simulink model "quadrotor_mellinger"  (R2024a)
settings: Solver=FixedStepAuto  StartTime=0.0  StopTime=30  FixedStep=0.0041667  RelTol=1e-3
values from neighbouring files (symbols this model uses):
  air_density = 1.229    [main2.m]    (also in param_set.m)
  bias_acc = task_bias_acc(task_id)    [main2.m]    (also in param_set.m = (-1+2*rand)*20/1000)
  bias_gyro = task_bias_gyro(task_id)    [main2.m]    (also in param_set.m = (-1+2*rand)*1)
  cf_mass = ori_mass + mass_payload    (= 0.027)    [main2.m]    (also in param_set.m)
  complex_pulse = ismember(task_id, [7, 8])    [main2.m]    (also in param_set.m = 0)
  delay_coef_acc = 100    [main2.m]    (also in param_set.m)
  delay_coef_gyro = 230    [main2.m]    (also in param_set.m)
  delay_coef_motor = 50    [main2.m]    (also in param_set.m)
  g = 9.81    [main2.m]    (also in param_set.m)
  goal_pos = task_goal_pos(task_id, :)    [main2.m]    (also in param_set.m = [0, 0.01, 1])
  GRAVITY_FORCE = g * cf_mass    (= 0.26487)    [main2.m]    (also in param_set.m)
  Kd_lin = data_struct.Kd_lin    [generate_mat_files.m]    (also in main2.m = [0.3114; 0.3114; 1.1489]; param_set.m = [0.3114; 0.3114; 1.1489])
  Ki_lin = data_struct.Ki_lin    [generate_mat_files.m]    (also in main2.m = [0.0027; 0.0027; 0.2500]; param_set.m = [0.0027; 0.0027; 0.2500])
  Ki_rot = data_struct.Ki_rot    [generate_mat_files.m]    (also in main2.m = [-1.2303; -1.2303; 494.9237]; param_set.m = [-1.2303; -1.2303; 494.9237])
  Kp_lin = data_struct.Kp_lin    [generate_mat_files.m]    (also in main2.m = [0.4319; 0.4319; 2.5857]; param_set.m = [0.4319; 0.4319; 2.5857])
  Kr_rot = data_struct.Kr_rot    [generate_mat_files.m]    (also in main2.m = [70000.0; 70000.0; 60000.0]; param_set.m = [70000.0; 70000.0; 60000.0])
  Kw_rot = data_struct.Kw_rot    [generate_mat_files.m]    (also in main2.m = [20000.0; 20000.0; 12000.0]; param_set.m = [20000.0; 20000.0; 12000.0])
  MassThrust = 132000    [main2.m]    (also in param_set.m)
  Matrix_rpm_Ftau = [ ... (first row only)    [main2.m]    (also in param_set.m)
  MaxPWM = 65535    [main2.m]    (also in param_set.m)
  measure_switch = mod(task_id, 2) == 0    [main2.m]    (also in param_set.m = 0)
  MIXER_MATRIX = [ ... (first row only)    [main2.m]    (also in param_set.m = [      -0.5, -0.5, -1.0;      -0.5,  0.5,  1.0;       0.5,  )
  pressure = 101.3e3    (= 101300)    [main2.m]    (also in param_set.m)
  PWM2RPM_CONST = 4070.3    [main2.m]    (also in param_set.m)
  PWM2RPM_SCALE = 0.2685    [main2.m]    (also in param_set.m)
  Speed_Sound = 340    [main2.m]    (also in param_set.m)
  T_flip = eye(3)    [main2.m]    (also in param_set.m = [1,  0,  0;            0,  1,  0;            0,  0,  1])
  target_x_c = [1; 0; 0]    [main2.m]    (also in param_set.m)
  UINT16_MAX = 65535    [main2.m]    (also in param_set.m)
  Wind_phi = 0    [main2.m]    (also in param_set.m)
  Wind_theta = 0    [main2.m]    (also in param_set.m)
  WorkTemperature = 25    [main2.m]    (also in param_set.m)
undefined symbols (not defined in the file or in its folder): DiscIntNeverNeededParam
libraries: simulink x12, slctrl_linear x3, sharedtransform x2, matrix_library x2, dspmathops x2, shared6dof x1
settings Model: Creator=cxk  LastModifiedBy=18065
settings OptimizationCC: ReuseModelBlockBuffer=off
settings RTWCC: GPUComputeCapability=3.5

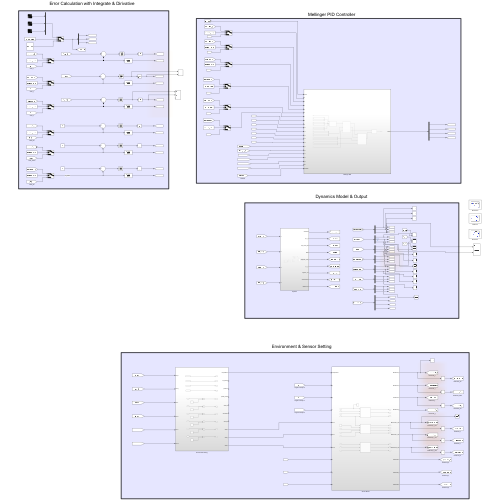
[thumbnail: Simulink's stored preview of the top-level diagram]
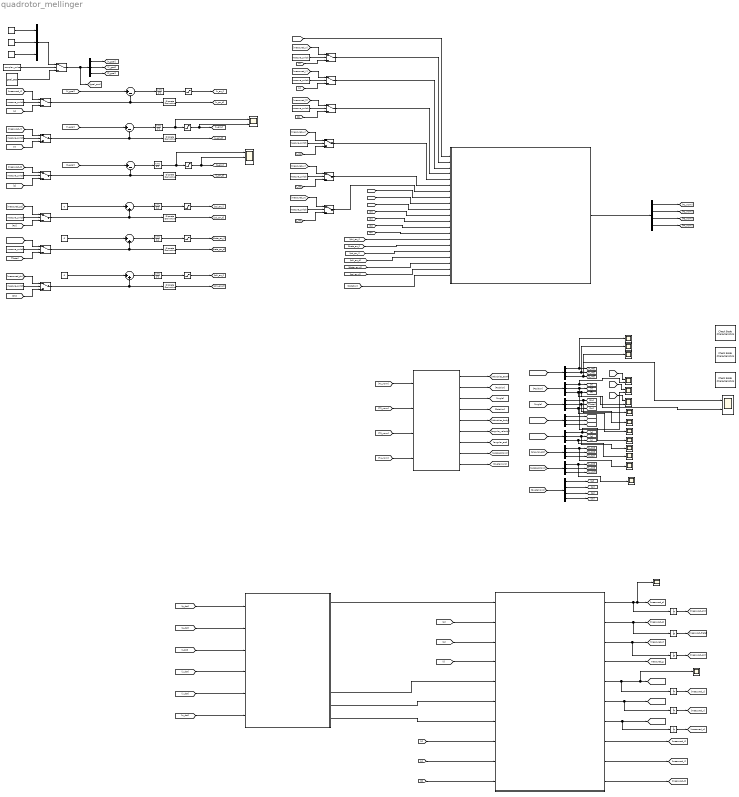
== system quadrotor_mellinger ==
  note: Mellinger PID Controller
  note: T1_norm
  note: Dynamics Model & Output
  note: Environment & Sensor Setting
  note: Error Calculation with Integrate & Dirivative
  Bode Plot : slctrl_linear/Check Bode  Characteristics  InstantiateOnLoad=on  SaveOperatingPoints=off  LinearizationIOs={'/Dynamic/From6', 1, 'outin', 'on', ''}  LinearizeAt=SnapshotTimes  SnapshotTimes=[0]  TriggerType=rising  SampleTime=auto  RateConversionMethod=zoh  PreWarpFreq=10  UseExactDelayModel=off  UseFullBlockNameLabels=off  UseBusSignalLabels=off  enabled=on  stopWhenAssertionFail=off  export=off  ViewDlgPos=[631 545 942 590]  OpenViewOnLoad=on  LaunchViewOnOpen=off  FrequencyUnits=rad/s  MagnitudeUnits=dB  PhaseUnits=deg  TimeUnits=seconds  EnableUpperBound=off  UpperBoundFrequencies=[]  UpperBoundMagnitudes=[]  EnableLowerBound=off  LowerBoundFrequencies=[]  LowerBoundMagnitudes=[]
      settings: LibrarySourceBlock=slctrlblks/Linear Analysis Plots/Bode Plot  SaveToWorkspace=off  SaveName=sys
  Bode Plot1 : slctrl_linear/Check Bode  Characteristics  InstantiateOnLoad=on  SaveOperatingPoints=off  LinearizationIOs={'/Dynamic/From6', 1, 'outin', 'on', ''}  LinearizeAt=SnapshotTimes  SnapshotTimes=[0]  TriggerType=rising  SampleTime=auto  RateConversionMethod=zoh  PreWarpFreq=10  UseExactDelayModel=off  UseFullBlockNameLabels=off  UseBusSignalLabels=off  enabled=on  stopWhenAssertionFail=off  export=off  ViewDlgPos=[1581 545.666666666667 957 589.333333333333]  OpenViewOnLoad=on  LaunchViewOnOpen=off  FrequencyUnits=rad/s  MagnitudeUnits=dB  PhaseUnits=deg  TimeUnits=seconds  EnableUpperBound=off  UpperBoundFrequencies=[]  UpperBoundMagnitudes=[]  EnableLowerBound=off  LowerBoundFrequencies=[]  LowerBoundMagnitudes=[]
      settings: LibrarySourceBlock=slctrlblks/Linear Analysis Plots/Bode Plot  SaveToWorkspace=off  SaveName=sys
  Bode Plot3 : slctrl_linear/Check Bode  Characteristics  InstantiateOnLoad=on  SaveOperatingPoints=off  LinearizationIOs={'/Dynamic/Sum', 1, 'outin', 'on', ''}  LinearizeAt=SnapshotTimes  SnapshotTimes=[0]  TriggerType=rising  SampleTime=auto  RateConversionMethod=zoh  PreWarpFreq=10  UseExactDelayModel=off  UseFullBlockNameLabels=off  UseBusSignalLabels=off  enabled=on  stopWhenAssertionFail=off  export=off  ViewDlgPos=[687.666666666667 401 778.666666666667 390]  OpenViewOnLoad=on  LaunchViewOnOpen=off  FrequencyUnits=rad/s  MagnitudeUnits=dB  PhaseUnits=deg  TimeUnits=seconds  EnableUpperBound=off  UpperBoundFrequencies=[]  UpperBoundMagnitudes=[]  EnableLowerBound=off  LowerBoundFrequencies=[]  LowerBoundMagnitudes=[]
      settings: LibrarySourceBlock=slctrlblks/Linear Analysis Plots/Bode Plot  SaveToWorkspace=off  SaveName=sys
  Constant : Constant  Value=goal_pos
  Constant1 : Constant  Value=0
  Constant{4..15} (12 alike) : Constant  Value=measure_switch
  Constant16 : Constant  Value=complex_pulse
  Constant2 : Constant  Value=0
  Constant3 : Constant  Value=0
  Demux{,1..4,6..7,9} (8 alike) : Demux  Outputs=3
  Demux10 : Demux
  Demux8 : Demux
  Discrete Derivative{,1..5} (6 alike) : simulink/Discrete/Discrete Derivative  gainval=1.0  ICPrevScaledInput=0.0  OutMin=[]  OutMax=[]  OutDataType=fixdt(1, 16)  OutScaling=2^-10  DoSatur=off
  Discrete-Time Integrator{,1..5} (6 alike) : DiscreteIntegrator  SampleTime=-1  ICPrevOutput=DiscIntNeverNeededParam  ICPrevScaledInput=DiscIntNeverNeededParam
  Dynamic : Subsystem
  Environment Setting : Subsystem
  Integrator{,1..5} (6 alike) : Integrator
  Mellinger PID : Subsystem
  Mux9 : Mux  Inputs=3
  Repeating Sequence1 : simulink/Sources/Repeating Sequence  rep_seq_t="[0 5 10  15 20 25 29]"  rep_seq_y=[0.05 0.05 2 2 -2 -2 0.05 ]
  Repeating Sequence2 : simulink/Sources/Repeating Sequence  rep_seq_t="[0 5 7  13 16 20 25 29]"  rep_seq_y=[0.05 0.05 1.68 1.68 -0.68 -0.68 0.05 0.05 ]
  Repeating Sequence3 : simulink/Sources/Repeating Sequence  rep_seq_t="[0 5 10  15 20 25 29]"  rep_seq_y=[0.05 0.05 2 2 -2 -2 0.05 ]
  Saturation : Saturate  UpperLimit=2  LowerLimit=-2
  Saturation1 : Saturate  UpperLimit=2  LowerLimit=-2
  Saturation2 : Saturate  UpperLimit=0.15  LowerLimit=-0.15
  Saturation3 : Saturate  UpperLimit=1  LowerLimit=-1
  Saturation4 : Saturate  UpperLimit=1  LowerLimit=-1
  Saturation5 : Saturate  UpperLimit=1  LowerLimit=-1
  Scope{,1..2,18,20} (5 alike) : Scope  NumInputPorts=2
  Scope{4..12,14,16..17,19} (13 alike) : Scope
  Scope15 : Scope  NumInputPorts=3
  Sensor Model : Subsystem
  Sum : Sum  Inputs=|+-
  Sum1 : Sum  Inputs=|+-
  Sum2 : Sum  Inputs=|+-
  Sum3 : Sum  Inputs=|++
  Sum4 : Sum  Inputs=|++
  Sum5 : Sum  Inputs=|++
  Switch{,1..11} (12 alike) : Switch  Criteria=u2 ~= 0  SaturateOnIntegerOverflow=off  InputSameDT=off
  Switch12 : Switch  Criteria=u2 > Threshold  SaturateOnIntegerOverflow=off  InputSameDT=off
  tag scope: measured_g=global
  wires:
  [T1_norm] -> Dynamic/1(In1)
  [T2_norm] -> Dynamic/2(In2)
  [T3_norm] -> Dynamic/3(In3)
  [T4_norm] -> Dynamic/4(In4)
  Dynamic/1(Velocities) -> [Velocities_earth]
  Dynamic/2(X_Y_Z) -> [Position]
  Dynamic/3(Phi_Theta_Psi) -> [Angle]
  Dynamic/4(DCM) -> [Rotation]
  Dynamic/5(Velocities_body) -> [Velocities_body]
  Dynamic/6(p_q_r) -> [angular_velocity]
  Dynamic/7(angular_acc) -> [angular_acc]
  Dynamic/8(Accelerations) -> [Accelerations]
  [Velocities_earth] -> Demux/1
  [Position] -> Demux1/1
  [Angle] -> Demux2/1
  [Accelerations] -> Demux7/1
  [angular_acc] -> Demux6/1
  [angular_velocity] -> Demux4/1
  [Velocities_body] -> Demux3/1
  Demux1/1 -> Scope/2, [X]
  Demux3/1 -> [Vx_Body]
  Demux3/2 -> [Vy_Body]
  Demux3/3 -> [Vz_Body]
  Demux6/1 -> Scope16/1, [p_dot]
  Demux6/2 -> [q_dot]
  Demux6/3 -> [r_dot]
  Demux7/1 -> Scope19/1, [u_dot]
  Demux7/2 -> [v_dot]
  Demux7/3 -> [w_dot]
  Dynamic/9(Quatenions) -> [Quatenions]
  [Quatenions] -> Demux8/1
  Demux8/1 -> [qr]
  Demux8/2 -> [qi]
  Demux9/1 -> [X_goal]
  Demux9/2 -> [Y_goal]
  Demux9/3 -> [Z_goal]
  [X_goal] -> Sum/1
  Switch1/1 -> Sum/2, Discrete Derivative2/1
  Saturation/1 -> [x_err_i]
  Discrete Derivative2/1 -> [x_err_d]
  [Y_goal] -> Sum1/1
  Switch/1 -> Sum1/2, Discrete Derivative1/1
  Discrete Derivative1/1 -> [y_err_d]
  Saturation1/1 -> Scope18/2, [y_err_i]
  [Z_goal] -> Sum2/1
  Switch2/1 -> Sum2/2, Discrete Derivative/1
  Sum2/1 -> Discrete-Time Integrator/1
  Saturation2/1 -> Scope15/2, [z_err_i]
  Saturation4/1 -> [theta_err_i]
  Constant3/1 -> Sum3/1
  Discrete Derivative4/1 -> [phi_err_d]
  Switch5/1 -> Sum3/2, Discrete Derivative4/1
  Constant2/1 -> Sum4/1
  Switch4/1 -> Sum4/2, Discrete Derivative5/1
  Discrete Derivative3/1 -> [psi_err_d]
  Saturation5/1 -> [psi_err_i]
  Switch3/1 -> Sum5/2, Discrete Derivative3/1
  Constant1/1 -> Sum5/1
  Saturation3/1 -> [phi_err_i]
  Demux10/2 -> [T2_norm]
  Demux10/4 -> [T4_norm]
  Demux10/3 -> [T3_norm]
  Switch9/1 -> Mellinger PID/2(In1)
  Switch10/1 -> Mellinger PID/3(In2)
  Switch11/1 -> Mellinger PID/4(In3)
  Switch6/1 -> Mellinger PID/5(In4)
  Switch8/1 -> Mellinger PID/6(In5)
  Switch7/1 -> Mellinger PID/7(In6)
  [x_err_i] -> Mellinger PID/8(In7)
  [y_err_i] -> Mellinger PID/9(In8)
  [z_err_i] -> Mellinger PID/10(In9)
  [qr] -> Mellinger PID/11(In10)
  [qi] -> Mellinger PID/12(In11)
  [qj] -> Mellinger PID/13(In12)
  [qk] -> Mellinger PID/14(In13)
  [phi_err_i] -> Mellinger PID/15(In14)
  [theta_err_i] -> Mellinger PID/16(In15)
  [psi_err_i] -> Mellinger PID/17(In16)
  [phi_err_d] -> Mellinger PID/18(In17)
  [theta_err_d] -> Mellinger PID/19(In18)
  [psi_err_d] -> Mellinger PID/20(In19)
  Mellinger PID/1(PWM) -> Demux10/1
  Demux10/1 -> [T1_norm]
  Demux8/3 -> [qj]
  Demux1/2 -> Scope1/2, [Y]
  Demux1/3 -> Scope2/2, Scope20/2, [Z]
  Demux2/2 -> Scope8/1, [Theta]
  Demux2/3 -> Scope9/1, [Psi]
  Demux4/3 -> Scope12/1, [r]
  Demux8/4 -> [qk]
  Demux2/1 -> [Phi], Scope4/1
  Demux4/1 -> Scope10/1, [p]
  Discrete Derivative/1 -> [z_err_d]
  Discrete-Time Integrator/1 -> Scope15/1, Saturation2/1
  Sum1/1 -> Discrete-Time Integrator1/1
  Discrete-Time Integrator1/1 -> Scope18/1, Saturation1/1
  Sum/1 -> Discrete-Time Integrator2/1
  Discrete-Time Integrator2/1 -> Saturation/1
  Sum5/1 -> Discrete-Time Integrator3/1
  Discrete-Time Integrator3/1 -> Saturation5/1
  Sum4/1 -> Discrete-Time Integrator4/1
  Discrete-Time Integrator4/1 -> Saturation4/1
  Sum3/1 -> Discrete-Time Integrator5/1
  Discrete-Time Integrator5/1 -> Saturation3/1
  Discrete Derivative5/1 -> [theta_err_d]
  Demux4/2 -> Scope11/1, [q]
  [Rotation] -> Mellinger PID/21(Rotation)
  Environment Setting/1(temperature) -> Sensor Model/1(Temperature)
  Environment Setting/8(wind x) -> Sensor Model/5(dot u)
  Environment Setting/9(wind y) -> Sensor Model/6(dot v)
  Environment Setting/10(wind z) -> Sensor Model/7(dot w)
  [p_dot] -> Environment Setting/1(dot p)
  [q_dot] -> Environment Setting/2("dot q ")
  [r_dot] -> Environment Setting/3(dot r)
  [u_dot] -> Environment Setting/4(dot u)
  [v_dot] -> Environment Setting/5(dot v)
  [w_dot] -> Environment Setting/6(dot w)
  Sensor Model/4(Measured g) -> [measured_g]
  Sensor Model/5(Measured u_dot) -> Scope17/1, [measured_u_dot], Integrator/1
  Sensor Model/6(Measured v_dot) -> Integrator1/1, [measured_v_dot]
  Sensor Model/7(Measured w_dot) -> Integrator2/1, [measured_w_dot]
  Constant4/1 -> Switch/2
  Constant5/1 -> Switch1/2
  Constant6/1 -> Switch2/2
  Constant7/1 -> Switch3/2
  Constant8/1 -> Switch4/2
  Constant9/1 -> Switch5/2
  [X] -> Switch1/3
  [Y] -> Switch/3
  [Z] -> Switch2/3
  [Psi] -> Switch3/3
  [Theta] -> Switch4/3
  [Phi] -> Switch5/3
  Constant10/1 -> Switch6/2
  [X_Vel] -> Switch6/3
  Constant11/1 -> Switch7/2
  Constant12/1 -> Switch8/2
  [Y_Vel] -> Switch8/3
  [Z_Vel] -> Switch7/3
  [measured_u] -> Switch6/1
  [measured_v] -> Switch8/1
  [measured_w] -> Switch7/1
  Sensor Model/1(Measured p) -> Integrator3/1, Scope14/1, [measured_p]
  Sensor Model/2(Measured q) -> Integrator4/1, [measured_q]
  Sensor Model/3(Measured r) -> Integrator5/1, [measured_r]
  [measured_psi] -> Switch3/1
  [measured_theta] -> Switch4/1
  [measured_phi] -> Switch5/1
  Constant13/1 -> Switch9/2
  Constant14/1 -> Switch10/2
  Constant15/1 -> Switch11/2
  [X] -> Switch9/3
  [Y] -> Switch10/3
  [Z] -> Switch11/3
  [X] -> Sensor Model/8(x)
  [Y] -> Sensor Model/9(y)
  [Z] -> Sensor Model/10(z)
  Sensor Model/8(Measured x) -> [measured_X]
  Sensor Model/9(Measured y) -> [measured_Y]
  Sensor Model/10(Measured z) -> [measured_Z]
  [measured_X] -> Switch1/1
  [measured_Y] -> Switch/1
  [measured_Z] -> Switch2/1
  [measured_X] -> Switch9/1
  [measured_Y] -> Switch10/1
  [measured_Z] -> Switch11/1
  [p] -> Sensor Model/2(p)
  [q] -> Sensor Model/3(q)
  [r] -> Sensor Model/4(r)
  Demux/1 -> Scope5/1, [X_Vel]
  Demux/2 -> Scope6/1, [Y_Vel]
  Demux/3 -> Scope20/1, [Z_Vel], Scope7/1
  Integrator3/1 -> [measured_phi]
  Integrator4/1 -> [measured_theta]
  Integrator5/1 -> [measured_psi]
  Integrator/1 -> [measured_u]
  Integrator1/1 -> [measured_v]
  Integrator2/1 -> [measured_w]
  Repeating Sequence2/1 -> Mux9/3
  [goal_pos] -> Mellinger PID/1(Goal)
  Switch12/1 -> [goal_pos], Demux9/1
  Repeating Sequence3/1 -> Mux9/1
  Repeating Sequence1/1 -> Mux9/2
  [Z_goal] -> Scope2/1
  [Y_goal] -> Scope1/1
  [X_goal] -> Scope/1
  Mux9/1 -> Switch12/1
  Constant/1 -> Switch12/3
  Constant16/1 -> Switch12/2

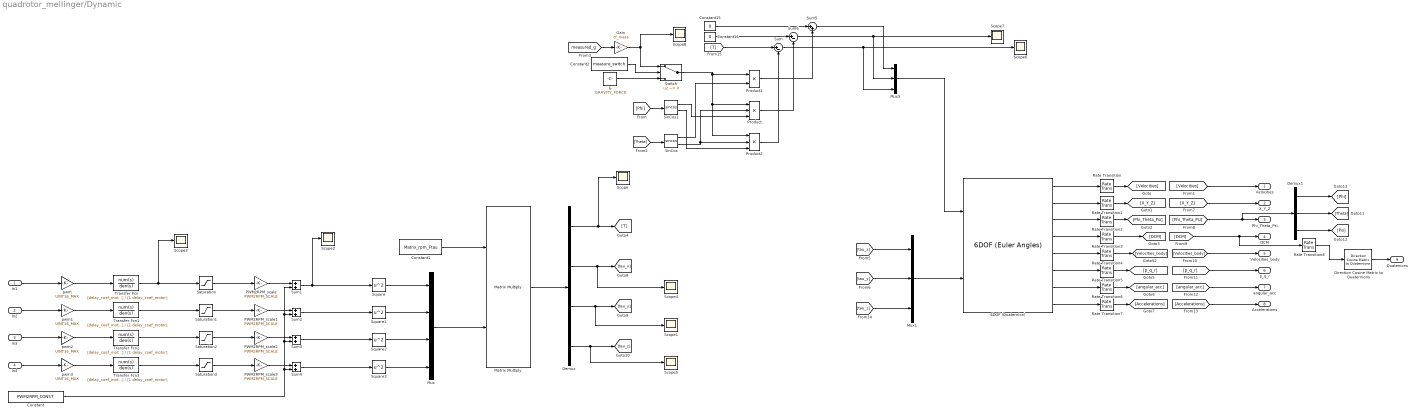
== system quadrotor_mellinger/Dynamic ==
  In1 : Inport
  In2 : Inport  Port=2
  In3 : Inport  Port=3
  In4 : Inport  Port=4
  6DOF (Quaternion) : shared6dof/6DOF (Euler Angles)  units=Metric (MKS)  mtype=Fixed  rep=Quaternion  xme_0=init_pos  Vm_0=init_vel  eul_0=init_ang  pm_0=[0 0 0]  mass_0=cf_mass  mass_e=0.5  mass_f=2.0  inertia=inertia  inertia_e=eye(3)  inertia_f=2*eye(3)  k_quat=1.0  vre_flag=on  abi_flag=off  aMode=0  xme_statename=''  Vm_statename=''  eul_statename=''  quat_statename=''  pm_statename=''  mass_statename=''
      settings: LibrarySourceBlock=aerolib6dof2/6DOF (Quaternion)
  Constant : Constant  Value=PWM2RPM_CONST
  Constant1 : Constant  Value=Matrix_rpm_Ftau
  Constant15 : Constant  Value=0
  Constant16 : Constant  Value=0
  Constant2 : Constant  Value=measure_switch
  Demux : Demux
  Demux1 : Demux  Outputs=3
  Direction Cosine Matrix to Quaternions : sharedtransform/Direction Cosine Matrix  to Quaternions  aMode=0  action=None  tolerance=eps(2)
      settings: LibrarySourceBlock=|
      | aerolibtransform2/Direction Cosine Matrix
      | to Quaternions
  G : Constant  Value=GRAVITY_FORCE
  Gain : Gain  Gain=cf_mass
  Matrix Multiply : Product  Multiplication=Matrix(*)
  Mux : Mux
  Mux1 : Mux  Inputs=3
  Mux5 : Mux  Inputs=3
  PWM2RPM_scale{,1..3} (4 alike) : Gain  Gain=PWM2RPM_SCALE
  Product : Product  Inputs=3
  Product1 : Product
  Product2 : Product  Inputs=3
  Rate Transition{,1..8} (9 alike) : RateTransition  OutPortSampleTimeOpt=Inherit  OutPortSampleTime=Ts
  Saturation{,1..3} (4 alike) : Saturate  UpperLimit=MaxPWM  LowerLimit=0
  Scope{,1..8} (9 alike) : Scope
  SinCos : Trigonometry  Operator=sincos
  SinCos1 : Trigonometry  Operator=sincos
  Square{,1..3} (4 alike) : Math  Operator=square
  Sum : Sum  Inputs=|+-
  Sum{1..4} (4 alike) : Sum
  Sum5 : Sum  Inputs=|++
  Sum6 : Sum  Inputs=|+-
  Switch : Switch  Criteria=u2 ~= 0  SaturateOnIntegerOverflow=off  InputSameDT=off
  Transfer Fcn{,1..3} (4 alike) : TransferFcn  Numerator=[delay_coef_motor]  Denominator=[1 delay_coef_motor]
  pwm{,1..3} (4 alike) : Gain  Gain=UINT16_MAX
  Velocities : Outport
  X_Y_Z : Outport  Port=2
  Phi_Theta_Psi : Outport  Port=3
  DCM : Outport  Port=4
  Velocities_body : Outport  Port=5
  p_q_r : Outport  Port=6
  angular_acc : Outport  Port=7
  Accelerations : Outport  Port=8
  Quatenions : Outport  Port=9
  wires:
  Rate Transition3/1 -> [DCM]
  Matrix Multiply/1 -> Demux/1
  Rate Transition6/1 -> [angular_acc]
  Rate Transition/1 -> [Velocities]
  [p_q_r] -> p_q_r/1
  [Velocities_body] -> Velocities_body/1
  [Phi_Theta_Psi] -> Demux1/1, Phi_Theta_Psi/1
  [tau_x] -> Mux1/1
  6DOF (Quaternion)/4 -> Rate Transition3/1
  Constant1/1 -> Matrix Multiply/1
  Demux/2 -> Scope4/1, [tau_x]
  Rate Transition5/1 -> [p_q_r]
  Rate Transition7/1 -> [Accelerations]
  Rate Transition1/1 -> [X_Y_Z]
  Rate Transition2/1 -> [Phi_Theta_Psi]
  Square1/1 -> Mux/2
  Demux/1 -> Scope/1, [T]
  Square3/1 -> Mux/4
  Mux/1 -> Matrix Multiply/2
  [Velocities] -> Velocities/1
  Rate Transition4/1 -> [Velocities_body]
  Square/1 -> Mux/1
  [DCM] -> Rate Transition8/1, DCM/1
  [X_Y_Z] -> X_Y_Z/1
  [Accelerations] -> Accelerations/1
  Demux/4 -> Scope5/1, [tau_z]
  [angular_acc] -> angular_acc/1
  Square2/1 -> Mux/3
  Demux/3 -> Scope1/1, [tau_y]
  Rate Transition8/1 -> Direction Cosine Matrix to Quaternions/1
  Direction Cosine Matrix to Quaternions/1 -> Quatenions/1
  Sum/1 -> Mux5/3, Scope6/1
  PWM2RPM_scale/1 -> Sum1/1
  Constant/1 -> Sum4/2, Sum3/2, Sum2/2, Sum1/2
  PWM2RPM_scale1/1 -> Sum2/1
  PWM2RPM_scale2/1 -> Sum3/1
  PWM2RPM_scale3/1 -> Sum4/1
  Sum2/1 -> Square1/1
  Sum1/1 -> Scope2/1, Square/1
  Sum3/1 -> Square2/1
  Sum4/1 -> Square3/1
  Saturation/1 -> PWM2RPM_scale/1
  Saturation1/1 -> PWM2RPM_scale1/1
  Saturation2/1 -> PWM2RPM_scale2/1
  Saturation3/1 -> PWM2RPM_scale3/1
  In4/1 -> pwm3/1
  pwm3/1 -> Transfer Fcn3/1
  In3/1 -> pwm2/1
  pwm2/1 -> Transfer Fcn2/1
  In2/1 -> pwm1/1
  pwm1/1 -> Transfer Fcn1/1
  In1/1 -> pwm/1
  pwm/1 -> Transfer Fcn/1
  Transfer Fcn/1 -> Scope3/1, Saturation/1
  Transfer Fcn1/1 -> Saturation1/1
  Transfer Fcn2/1 -> Saturation2/1
  Transfer Fcn3/1 -> Saturation3/1
  Demux1/2 -> [Theta]
  Demux1/3 -> [Psi]
  Demux1/1 -> [Phi]
  [Theta] -> SinCos/1
  [Phi] -> SinCos1/1
  Sum6/1 -> Mux5/2, Scope7/1
  Sum5/1 -> Mux5/1
  SinCos/1 -> Product1/2
  Product1/1 -> Sum5/2
  SinCos/2 -> Product2/2, Product/2
  SinCos1/2 -> Product2/3
  SinCos1/1 -> Product/3
  Product2/1 -> Sum/2
  Product/1 -> Sum6/2
  Constant16/1 -> Sum6/1
  Constant15/1 -> Sum5/1
  Mux1/1 -> 6DOF (Quaternion)/2
  Mux5/1 -> 6DOF (Quaternion)/1
  6DOF (Quaternion)/2 -> Rate Transition1/1
  6DOF (Quaternion)/1 -> Rate Transition/1
  6DOF (Quaternion)/3 -> Rate Transition2/1
  6DOF (Quaternion)/5 -> Rate Transition4/1
  6DOF (Quaternion)/7 -> Rate Transition6/1
  6DOF (Quaternion)/8 -> Rate Transition7/1
  [tau_y] -> Mux1/2
  [tau_z] -> Mux1/3
  G/1 -> Switch/3
  [measured_g] -> Gain/1
  Constant2/1 -> Switch/2
  [T] -> Sum/1
  Switch/1 -> Product1/1, Product2/1, Product/1
  Gain/1 -> Switch/1, Scope8/1
  6DOF (Quaternion)/6 -> Rate Transition5/1

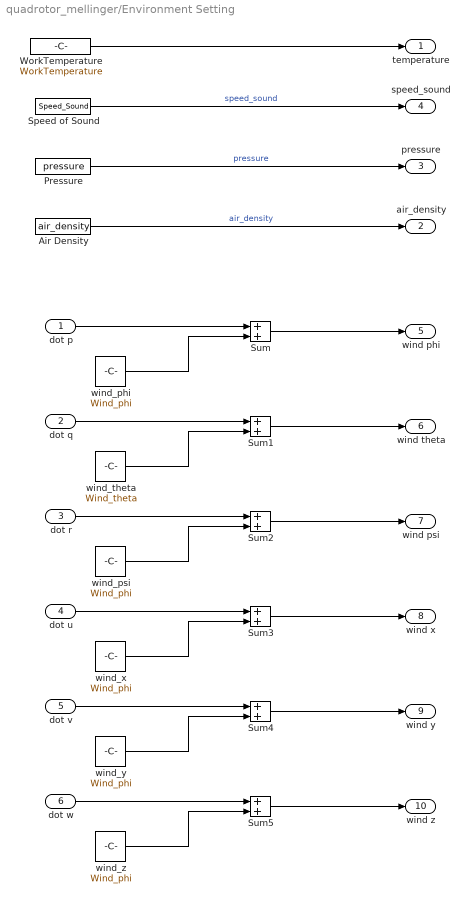
== system quadrotor_mellinger/Environment Setting ==
  dot p : Inport
  "dot q " : Inport  Port=2
  dot r : Inport  Port=3
  dot u : Inport  Port=4
  dot v : Inport  Port=5
  dot w : Inport  Port=6
  Air Density : Constant  Value=air_density
  Pressure : Constant  Value=pressure
  Speed of Sound : Constant  Value=Speed_Sound
  Sum{,1..5} (6 alike) : Sum
  WorkTemperature : Constant  Value=WorkTemperature
  wind_phi : Constant  Value=Wind_phi
  wind_psi : Constant  Value=Wind_phi
  wind_theta : Constant  Value=Wind_theta
  wind_x : Constant  Value=Wind_phi
  wind_y : Constant  Value=Wind_phi
  wind_z : Constant  Value=Wind_phi
  temperature : Outport
  air_density : Outport  Port=2
  pressure : Outport  Port=3
  speed_sound : Outport  Port=4
  wind phi : Outport  Port=5
  wind theta : Outport  Port=6
  wind psi : Outport  Port=7
  wind x : Outport  Port=8
  wind y : Outport  Port=9
  wind z : Outport  Port=10
  wires:
  Air Density/1 -> air_density/1  "air_density"
  Speed of Sound/1 -> speed_sound/1  "speed_sound"
  WorkTemperature/1 -> temperature/1
  Pressure/1 -> pressure/1  "pressure"
  dot p/1 -> Sum/1
  Sum/1 -> wind phi/1
  wind_theta/1 -> Sum1/2
  Sum1/1 -> wind theta/1
  "dot q "/1 -> Sum1/1
  wind_psi/1 -> Sum2/2
  Sum2/1 -> wind psi/1
  dot r/1 -> Sum2/1
  wind_x/1 -> Sum3/2
  Sum3/1 -> wind x/1
  dot u/1 -> Sum3/1
  wind_y/1 -> Sum4/2
  Sum4/1 -> wind y/1
  dot v/1 -> Sum4/1
  Sum5/1 -> wind z/1
  dot w/1 -> Sum5/1
  wind_phi/1 -> Sum/2
  wind_z/1 -> Sum5/2

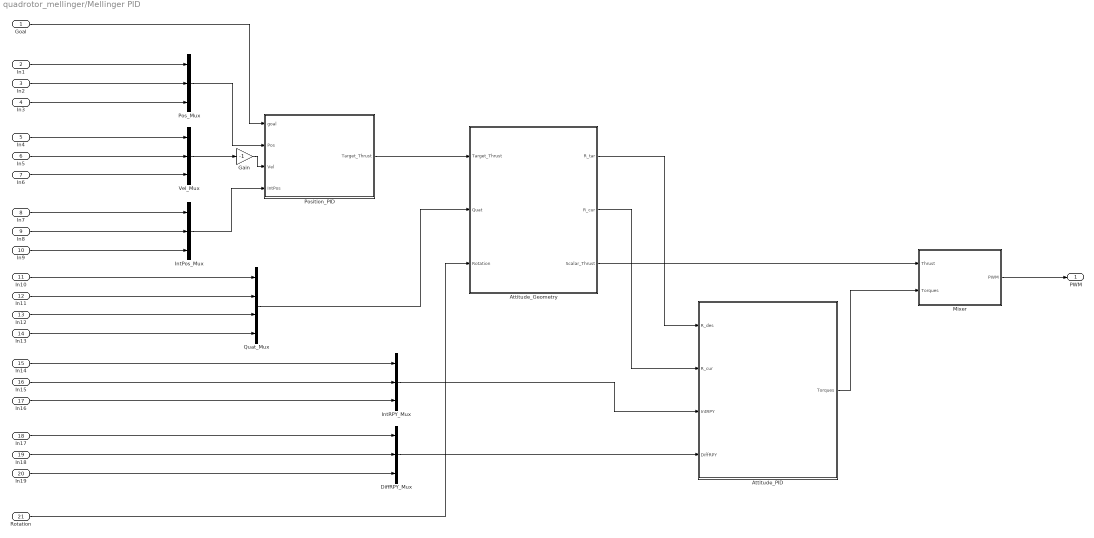
== system quadrotor_mellinger/Mellinger PID ==
  Goal : Inport
  In1 : Inport  Port=2
  In2 : Inport  Port=3
  In3 : Inport  Port=4
  In4 : Inport  Port=5
  In5 : Inport  Port=6
  In6 : Inport  Port=7
  In7 : Inport  Port=8
  In8 : Inport  Port=9
  In9 : Inport  Port=10
  In10 : Inport  Port=11
  In11 : Inport  Port=12
  In12 : Inport  Port=13
  In13 : Inport  Port=14
  In14 : Inport  Port=15
  In15 : Inport  Port=16
  In16 : Inport  Port=17
  In17 : Inport  Port=18
  In18 : Inport  Port=19
  In19 : Inport  Port=20
  Rotation : Inport  Port=21
  Attitude_Geometry : Subsystem
  Attitude_PID : Subsystem
  DiffRPY_Mux : Mux  Inputs=3
  Gain : Gain  Gain=-1
  IntPos_Mux : Mux  Inputs=3
  IntRPY_Mux : Mux  Inputs=3
  Mixer : Subsystem
  Pos_Mux : Mux  Inputs=3
  Position_PID : Subsystem
  Quat_Mux : Mux
  Vel_Mux : Mux  Inputs=3
  PWM : Outport
  wires:
  Attitude_Geometry/2(R_cur) -> Attitude_PID/2(R_cur)
  DiffRPY_Mux/1 -> Attitude_PID/4(DiffRPY)
  In17/1 -> DiffRPY_Mux/1
  In10/1 -> Quat_Mux/1
  Vel_Mux/1 -> Gain/1
  In3/1 -> Pos_Mux/3
  In9/1 -> IntPos_Mux/3
  Attitude_Geometry/3(Scalar_Thrust) -> Mixer/1(Thrust)
  In19/1 -> DiffRPY_Mux/3
  IntPos_Mux/1 -> Position_PID/4(IntPos)
  In15/1 -> IntRPY_Mux/2
  In7/1 -> IntPos_Mux/1
  In8/1 -> IntPos_Mux/2
  Quat_Mux/1 -> Attitude_Geometry/2(Quat)
  IntRPY_Mux/1 -> Attitude_PID/3(IntRPY)
  Pos_Mux/1 -> Position_PID/2(Pos)
  Attitude_PID/1(Torques) -> Mixer/2(Torques)
  Attitude_Geometry/1(R_tar) -> Attitude_PID/1(R_des)
  In11/1 -> Quat_Mux/2
  Position_PID/1(Target_Thrust) -> Attitude_Geometry/1(Target_Thrust)
  In18/1 -> DiffRPY_Mux/2
  In13/1 -> Quat_Mux/4
  In12/1 -> Quat_Mux/3
  In2/1 -> Pos_Mux/2
  In1/1 -> Pos_Mux/1
  In14/1 -> IntRPY_Mux/1
  In16/1 -> IntRPY_Mux/3
  In4/1 -> Vel_Mux/1
  In6/1 -> Vel_Mux/3
  In5/1 -> Vel_Mux/2
  Mixer/1(PWM) -> PWM/1
  Gain/1 -> Position_PID/3(Vel)
  Rotation/1 -> Attitude_Geometry/3(Rotation)
  Goal/1 -> Position_PID/1(goal)

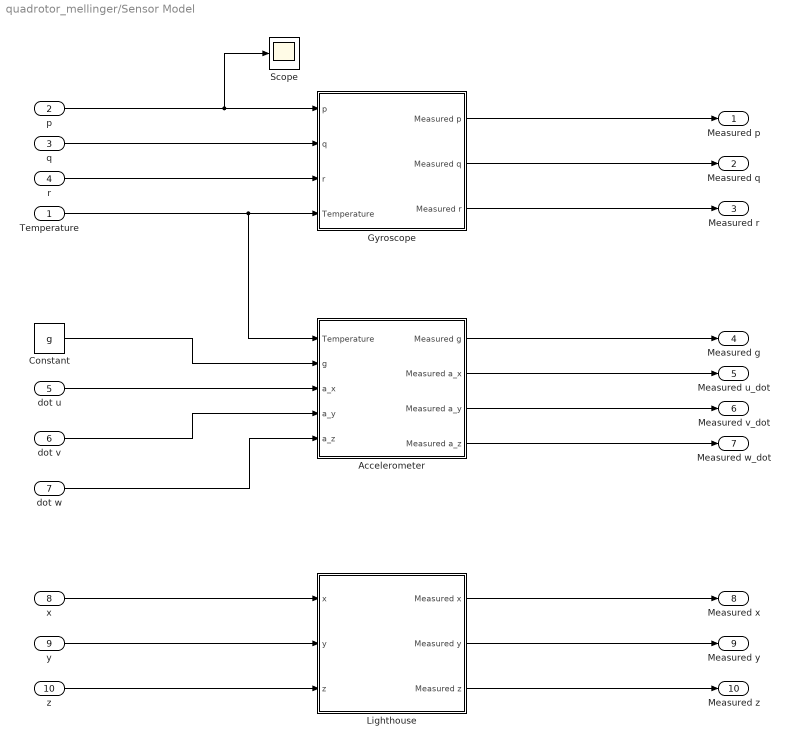
== system quadrotor_mellinger/Sensor Model ==
  Temperature : Inport
  p : Inport  Port=2
  q : Inport  Port=3
  r : Inport  Port=4
  dot u : Inport  Port=5
  dot v : Inport  Port=6
  dot w : Inport  Port=7
  x : Inport  Port=8
  y : Inport  Port=9
  z : Inport  Port=10
  Accelerometer : Subsystem
  Constant : Constant  Value=g
  Gyroscope : Subsystem
  Lighthouse : Subsystem
  Scope : Scope
  Measured p : Outport
  Measured q : Outport  Port=2
  Measured r : Outport  Port=3
  Measured g : Outport  Port=4
  Measured u_dot : Outport  Port=5
  Measured v_dot : Outport  Port=6
  Measured w_dot : Outport  Port=7
  Measured x : Outport  Port=8
  Measured y : Outport  Port=9
  Measured z : Outport  Port=10
  wires:
  Temperature/1 -> Accelerometer/1(Temperature), Gyroscope/4(Temperature)
  Gyroscope/1(Measured p) -> Measured p/1
  Gyroscope/2(Measured q) -> Measured q/1
  Gyroscope/3(Measured r) -> Measured r/1
  Constant/1 -> Accelerometer/2(g)
  dot u/1 -> Accelerometer/3(a_x)
  dot v/1 -> Accelerometer/4(a_y)
  dot w/1 -> Accelerometer/5(a_z)
  Accelerometer/1(Measured g) -> Measured g/1
  Accelerometer/2(Measured a_x) -> Measured u_dot/1
  Accelerometer/3(Measured a_y) -> Measured v_dot/1
  Accelerometer/4(Measured a_z) -> Measured w_dot/1
  p/1 -> Scope/1, Gyroscope/1(p)
  q/1 -> Gyroscope/2(q)
  r/1 -> Gyroscope/3(r)
  x/1 -> Lighthouse/1(x)
  y/1 -> Lighthouse/2(y)
  z/1 -> Lighthouse/3(z)
  Lighthouse/1(Measured x) -> Measured x/1
  Lighthouse/2(Measured y) -> Measured y/1
  Lighthouse/3(Measured z) -> Measured z/1

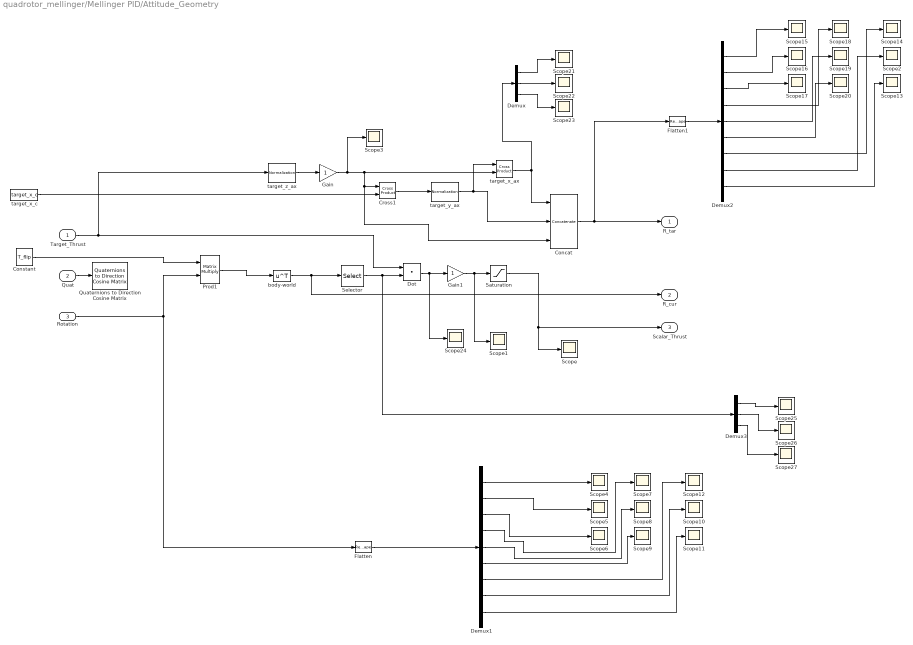
== system quadrotor_mellinger/Mellinger PID/Attitude_Geometry ==
  Target_Thrust : Inport
  Quat : Inport  Port=2
  Rotation : Inport  Port=3
  Concat : Concatenate  NumInputs=3  Mode=Multidimensional array  ConcatenateDimension=2
  Constant : Constant  Value=T_flip
  Cross1 : matrix_library/Cross Product
  Demux : Demux  Outputs=3
  Demux1 : Demux  Outputs=9
  Demux2 : Demux  Outputs=9
  Demux3 : Demux  Outputs=3
  Dot : DotProduct
  Flatten : Reshape
  Flatten1 : Reshape
  Gain : Gain
  Gain1 : Gain
  Prod1 : Product  Multiplication=Matrix(*)
  Quaternions to Direction Cosine Matrix : sharedtransform/Quaternions to  Direction Cosine Matrix  aMode=aMode
      settings: LibrarySourceBlock=|
      | aerolibtransform2/Quaternions to
      | Direction Cosine Matrix
  Saturation : Saturate  UpperLimit=Inf  LowerLimit=0
  Scope{,1..27} (28 alike) : Scope
  Selector : Selector  NumberOfDimensions=2  InputPortWidth=3  IndexOptions=Index vector (dialog),Index vector (dialog)  Indices=[1,2,3],3  OutputSizes=1,1
  body-world : Math  Operator=transpose
  target_x_ax : matrix_library/Cross Product
  target_x_c : Constant  Value=target_x_c
  target_y_ax : dspmathops/Normalization  NormType=2-norm  Bias=1e-12  NormOver=Each column  Dimension=1  roundingMode=Floor  overflowMode=off  accumDataTypeStr=Inherit: Same as product output  accumLastDataTypeStr=Inherit: Same as product output  outputDataTypeStr=Inherit: Same as product output  outputMin=[]  outputMax=[]  outputLastDataTypeStr=Inherit: Same as product output
  target_z_ax : dspmathops/Normalization  NormType=2-norm  Bias=1e-12  NormOver=Each column  Dimension=1  roundingMode=Floor  overflowMode=off  accumDataTypeStr=Inherit: Same as product output  accumLastDataTypeStr=Inherit: Same as product output  outputDataTypeStr=Inherit: Same as product output  outputMin=[]  outputMax=[]  outputLastDataTypeStr=Inherit: Same as product output
  R_tar : Outport
  R_cur : Outport  Port=2
  Scalar_Thrust : Outport  Port=3
  wires:
  Quat/1 -> Quaternions to Direction Cosine Matrix/1
  Target_Thrust/1 -> target_z_ax/1, Dot/1
  target_x_c/1 -> Cross1/2
  Cross1/1 -> target_y_ax/1
  target_y_ax/1 -> target_x_ax/1, Concat/2
  Saturation/1 -> Scope/1, Scalar_Thrust/1
  body-world/1 -> Selector/1, R_cur/1
  Demux1/8 -> Scope10/1
  Demux1/6 -> Scope9/1
  Demux1/9 -> Scope11/1
  Demux1/5 -> Scope8/1
  Demux1/3 -> Scope6/1
  Demux1/1 -> Scope4/1
  Demux1/4 -> Scope7/1
  Demux1/2 -> Scope5/1
  Flatten/1 -> Demux1/1
  Demux1/7 -> Scope12/1
  Flatten1/1 -> Demux2/1
  Demux2/8 -> Scope2/1
  Demux2/3 -> Scope17/1
  Demux2/9 -> Scope13/1
  Demux2/5 -> Scope19/1
  Demux2/1 -> Scope15/1
  Demux2/7 -> Scope14/1
  Demux2/6 -> Scope20/1
  Demux2/4 -> Scope18/1
  Concat/1 -> Flatten1/1, R_tar/1
  Demux2/2 -> Scope16/1
  target_x_ax/1 -> Demux/1, Concat/1
  Demux/1 -> Scope21/1
  Demux/3 -> Scope23/1
  Demux/2 -> Scope22/1
  target_z_ax/1 -> Gain/1
  Gain/1 -> Scope3/1, target_x_ax/2, Concat/3, Cross1/1
  Dot/1 -> Gain1/1, Scope24/1
  Constant/1 -> Prod1/1
  Selector/1 -> Demux3/1, Dot/2
  Demux3/1 -> Scope25/1
  Demux3/2 -> Scope26/1
  Demux3/3 -> Scope27/1
  Rotation/1 -> Flatten/1, Prod1/2
  Prod1/1 -> body-world/1
  Gain1/1 -> Scope1/1, Saturation/1

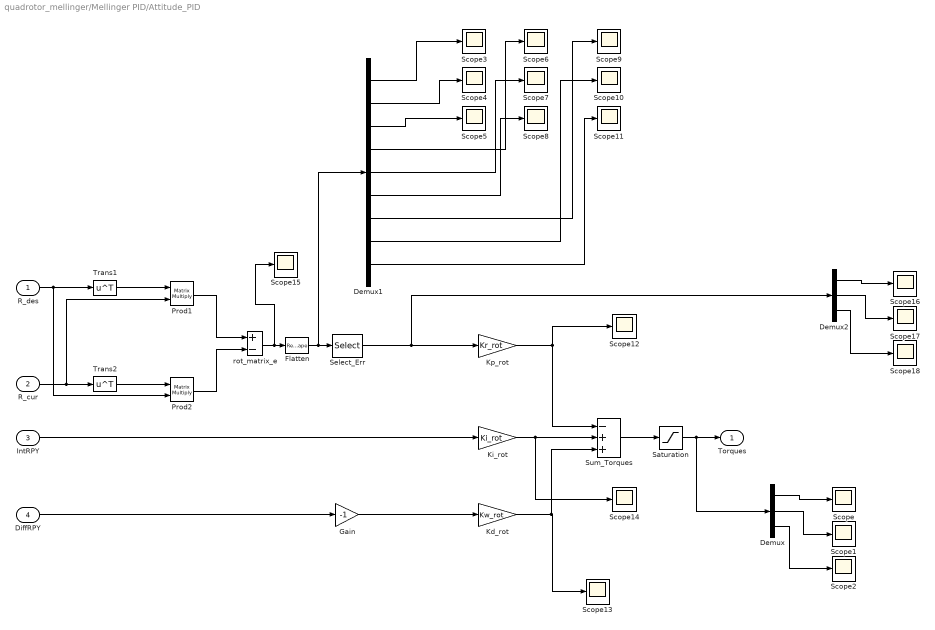
== system quadrotor_mellinger/Mellinger PID/Attitude_PID ==
  R_des : Inport
  R_cur : Inport  Port=2
  IntRPY : Inport  Port=3
  DiffRPY : Inport  Port=4
  Demux : Demux  Outputs=3
  Demux1 : Demux  Outputs=9
  Demux2 : Demux  Outputs=3
  Flatten : Reshape
  Gain : Gain  Gain=-1
  Kd_rot : Gain  Gain=Kw_rot
  Ki_rot : Gain  Gain=Ki_rot
  Kp_rot : Gain  Gain=Kr_rot
  Prod1 : Product  Multiplication=Matrix(*)
  Prod2 : Product  Multiplication=Matrix(*)
  Saturation : Saturate  UpperLimit=32000  LowerLimit=-32000
  Scope{,1..18} (19 alike) : Scope
  Select_Err : Selector  IndexOptions=Index vector (dialog)  Indices=[6 7 2]  OutputSizes=1
  Sum_Torques : Sum  Inputs=-++
  Trans1 : Math  Operator=transpose
  Trans2 : Math  Operator=transpose
  rot_matrix_e : Sum  Inputs=+-
  Torques : Outport
  wires:
  Trans1/1 -> Prod1/1
  R_cur/1 -> Prod1/2, Trans2/1
  Trans2/1 -> Prod2/1
  R_des/1 -> Prod2/2, Trans1/1
  Prod1/1 -> rot_matrix_e/1
  Prod2/1 -> rot_matrix_e/2
  rot_matrix_e/1 -> Scope15/1, Flatten/1
  Flatten/1 -> Demux1/1, Select_Err/1
  IntRPY/1 -> Ki_rot/1
  Kp_rot/1 -> Sum_Torques/1, Scope12/1
  Ki_rot/1 -> Sum_Torques/2, Scope14/1
  Kd_rot/1 -> Sum_Torques/3, Scope13/1
  Sum_Torques/1 -> Saturation/1
  Saturation/1 -> Demux/1, Torques/1
  DiffRPY/1 -> Gain/1
  Gain/1 -> Kd_rot/1
  Demux/1 -> Scope/1
  Demux/2 -> Scope1/1
  Demux/3 -> Scope2/1
  Demux1/1 -> Scope3/1
  Demux1/2 -> Scope4/1
  Demux1/3 -> Scope5/1
  Demux1/4 -> Scope6/1
  Demux1/5 -> Scope7/1
  Demux1/6 -> Scope8/1
  Demux1/7 -> Scope9/1
  Demux1/8 -> Scope10/1
  Demux1/9 -> Scope11/1
  Demux2/1 -> Scope16/1
  Select_Err/1 -> Demux2/1, Kp_rot/1
  Demux2/3 -> Scope18/1
  Demux2/2 -> Scope17/1

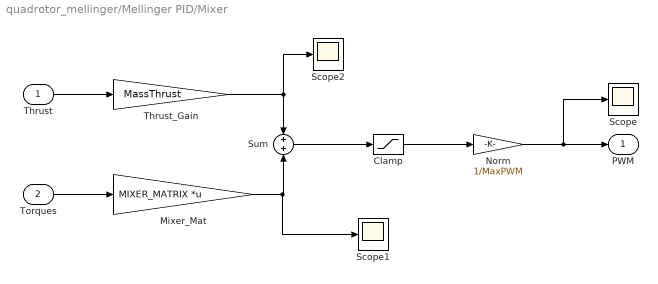
== system quadrotor_mellinger/Mellinger PID/Mixer ==
  Thrust : Inport
  Torques : Inport  Port=2
  Clamp : Saturate  UpperLimit=MaxPWM  LowerLimit=0
  Mixer_Mat : Gain  Gain=MIXER_MATRIX  Multiplication=Matrix(K*u)
  Norm : Gain  Gain=1/MaxPWM
  Scope : Scope
  Scope1 : Scope
  Scope2 : Scope
  Sum : Sum
  Thrust_Gain : Gain  Gain=MassThrust
  PWM : Outport
  wires:
  Thrust/1 -> Thrust_Gain/1
  Torques/1 -> Mixer_Mat/1
  Thrust_Gain/1 -> Sum/1, Scope2/1
  Mixer_Mat/1 -> Scope1/1, Sum/2
  Sum/1 -> Clamp/1
  Clamp/1 -> Norm/1
  Norm/1 -> Scope/1, PWM/1

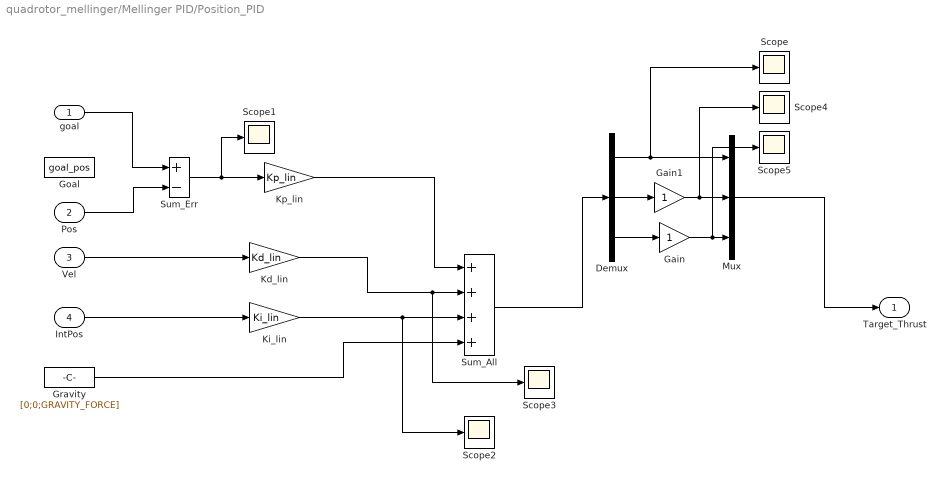
== system quadrotor_mellinger/Mellinger PID/Position_PID ==
  goal : Inport
  Pos : Inport  Port=2
  Vel : Inport  Port=3
  IntPos : Inport  Port=4
  Demux : Demux  Outputs=3
  Gain : Gain
  Gain1 : Gain
  Goal : Constant  Value=goal_pos
  Gravity : Constant  Value=[0;0;GRAVITY_FORCE]
  Kd_lin : Gain  Gain=Kd_lin
  Ki_lin : Gain  Gain=Ki_lin
  Kp_lin : Gain  Gain=Kp_lin
  Mux : Mux  Inputs=3
  Scope{,1..5} (6 alike) : Scope
  Sum_All : Sum  Inputs=++++
  Sum_Err : Sum  Inputs=+-
  Target_Thrust : Outport
  wires:
  Pos/1 -> Sum_Err/2
  Sum_Err/1 -> Scope1/1, Kp_lin/1
  Vel/1 -> Kd_lin/1
  IntPos/1 -> Ki_lin/1
  Ki_lin/1 -> Scope2/1, Sum_All/3
  Kd_lin/1 -> Scope3/1, Sum_All/2
  Demux/1 -> Scope/1, Mux/1
  Demux/2 -> Gain1/1
  Demux/3 -> Gain/1
  Sum_All/1 -> Demux/1
  Mux/1 -> Target_Thrust/1
  Gain/1 -> Mux/3, Scope5/1
  Gain1/1 -> Mux/2, Scope4/1
  Kp_lin/1 -> Sum_All/1
  Gravity/1 -> Sum_All/4
  goal/1 -> Sum_Err/1

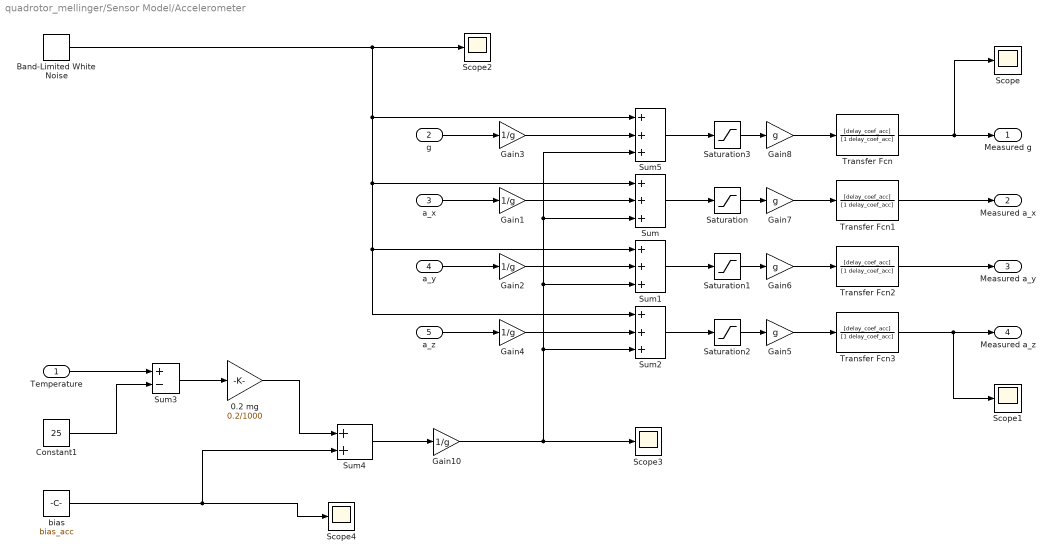
== system quadrotor_mellinger/Sensor Model/Accelerometer ==
  Temperature : Inport
  g : Inport  Port=2
  a_x : Inport  Port=3
  a_y : Inport  Port=4
  a_z : Inport  Port=5
  0.2 mg : Gain  Gain=0.2/1000
  Band-Limited White Noise : simulink/Sources/Band-Limited White Noise  Cov=[(160/g/1000000)^2]  Ts=0.0041667  seed=[23341]
  Constant1 : Constant  Value=25
  Gain{1..4,10} (5 alike) : Gain  Gain=1/g
  Gain{5..8} (4 alike) : Gain  Gain=g
  Saturation{,1..3} (4 alike) : Saturate  UpperLimit=6  LowerLimit=-6
  Scope{,1..4} (5 alike) : Scope
  Sum{,1..2,5} (4 alike) : Sum  Inputs=+++
  Sum3 : Sum  Inputs=+-
  Sum4 : Sum
  Transfer Fcn{,1..3} (4 alike) : TransferFcn  Numerator=[delay_coef_acc]  Denominator=[1 delay_coef_acc]
  bias : Constant  Value=bias_acc
  Measured g : Outport
  Measured a_x : Outport  Port=2
  Measured a_y : Outport  Port=3
  Measured a_z : Outport  Port=4
  wires:
  Saturation1/1 -> Gain6/1
  Saturation/1 -> Gain7/1
  a_y/1 -> Gain2/1
  0.2 mg/1 -> Sum4/1
  Temperature/1 -> Sum3/1
  a_x/1 -> Gain1/1
  Sum2/1 -> Saturation2/1
  Saturation2/1 -> Gain5/1
  a_z/1 -> Gain4/1
  Sum1/1 -> Saturation1/1
  bias/1 -> Scope4/1, Sum4/2
  Constant1/1 -> Sum3/2
  Sum/1 -> Saturation/1
  Sum3/1 -> 0.2 mg/1
  Sum5/1 -> Saturation3/1
  Sum4/1 -> Gain10/1
  Saturation3/1 -> Gain8/1
  g/1 -> Gain3/1
  Gain1/1 -> Sum/2
  Gain2/1 -> Sum1/2
  Gain3/1 -> Sum5/2
  Gain4/1 -> Sum2/2
  Gain5/1 -> Transfer Fcn3/1
  Gain6/1 -> Transfer Fcn2/1
  Gain7/1 -> Transfer Fcn1/1
  Gain8/1 -> Transfer Fcn/1
  Transfer Fcn/1 -> Scope/1, Measured g/1
  Transfer Fcn1/1 -> Measured a_x/1
  Transfer Fcn2/1 -> Measured a_y/1
  Transfer Fcn3/1 -> Scope1/1, Measured a_z/1
  Band-Limited White Noise/1 -> Sum2/1, Sum1/1, Sum/1, Sum5/1, Scope2/1
  Gain10/1 -> Sum5/3, Sum/3, Sum1/3, Sum2/3, Scope3/1

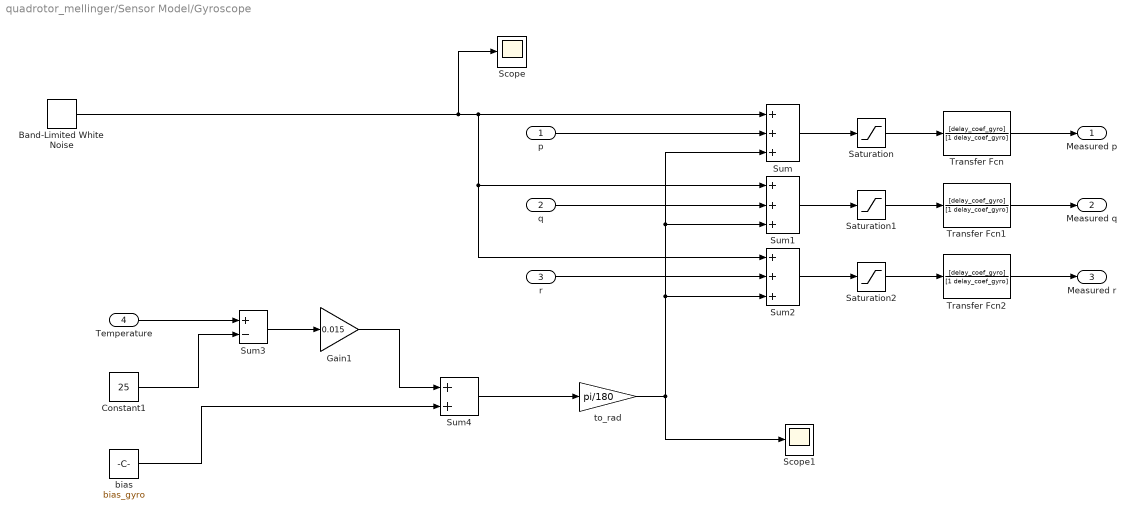
== system quadrotor_mellinger/Sensor Model/Gyroscope ==
  p : Inport
  q : Inport  Port=2
  r : Inport  Port=3
  Temperature : Inport  Port=4
  Band-Limited White Noise : simulink/Sources/Band-Limited White Noise  Cov=[(0.014/180*pi)^2]  Ts=0.0041667  seed=[23341]
  Constant1 : Constant  Value=25
  Gain1 : Gain  Gain=0.015
  Saturation : Saturate  UpperLimit=500  LowerLimit=-500
  Saturation1 : Saturate  UpperLimit=500  LowerLimit=-500
  Saturation2 : Saturate  UpperLimit=500  LowerLimit=-500
  Scope : Scope
  Scope1 : Scope
  Sum : Sum  Inputs=+++
  Sum1 : Sum  Inputs=+++
  Sum2 : Sum  Inputs=+++
  Sum3 : Sum  Inputs=+-
  Sum4 : Sum
  Transfer Fcn : TransferFcn  Numerator=[delay_coef_gyro]  Denominator=[1 delay_coef_gyro]
  Transfer Fcn1 : TransferFcn  Numerator=[delay_coef_gyro]  Denominator=[1 delay_coef_gyro]
  Transfer Fcn2 : TransferFcn  Numerator=[delay_coef_gyro]  Denominator=[1 delay_coef_gyro]
  bias : Constant  Value=bias_gyro
  to_rad : Gain  Gain=pi/180
  Measured p : Outport
  Measured q : Outport  Port=2
  Measured r : Outport  Port=3
  wires:
  Saturation1/1 -> Transfer Fcn1/1
  Saturation/1 -> Transfer Fcn/1
  q/1 -> Sum1/2
  Sum4/1 -> to_rad/1
  Gain1/1 -> Sum4/1
  Temperature/1 -> Sum3/1
  p/1 -> Sum/2
  Sum2/1 -> Saturation2/1
  Saturation2/1 -> Transfer Fcn2/1
  r/1 -> Sum2/2
  Sum1/1 -> Saturation1/1
  bias/1 -> Sum4/2
  Constant1/1 -> Sum3/2
  Sum/1 -> Saturation/1
  Sum3/1 -> Gain1/1
  to_rad/1 -> Scope1/1, Sum1/3, Sum/3, Sum2/3
  Band-Limited White Noise/1 -> Scope/1, Sum2/1, Sum1/1, Sum/1
  Transfer Fcn/1 -> Measured p/1
  Transfer Fcn1/1 -> Measured q/1
  Transfer Fcn2/1 -> Measured r/1

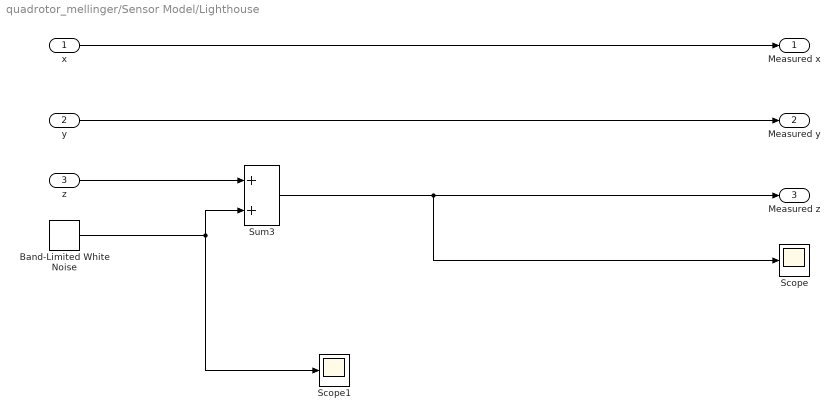
== system quadrotor_mellinger/Sensor Model/Lighthouse ==
  x : Inport
  y : Inport  Port=2
  z : Inport  Port=3
  Band-Limited White Noise : simulink/Sources/Band-Limited White Noise  Cov=[0.000005]  Ts=0.0041667  seed=[23341]
  Scope : Scope
  Scope1 : Scope
  Sum3 : Sum
  Measured x : Outport
  Measured y : Outport  Port=2
  Measured z : Outport  Port=3
  wires:
  x/1 -> Measured x/1
  y/1 -> Measured y/1
  z/1 -> Sum3/1
  Band-Limited White Noise/1 -> Sum3/2, Scope1/1
  Sum3/1 -> Scope/1, Measured z/1
